simulink model "BMS_CurrentLimitsCalc_COM_Harness_MIL"  (R2022b)
settings: configuration reference "BMS_Sw_CodeGenConfig" (kept outside this file)
model workspace: external: MAT-File H:\0\New MAAM\10 - MBD\Battary Management System\SWE.3 CDD\DataTypes\Data_Script.mat (data not in the file)
undefined symbols (not defined in the file): BATT, Schedule
settings Model: DataDictionary=BMS_Arch_DD.sldd  Creator=MAAM  LastModifiedBy=MAAM
settings ConfigSetRef: SourceName=BMS_Sw_CodeGenConfig

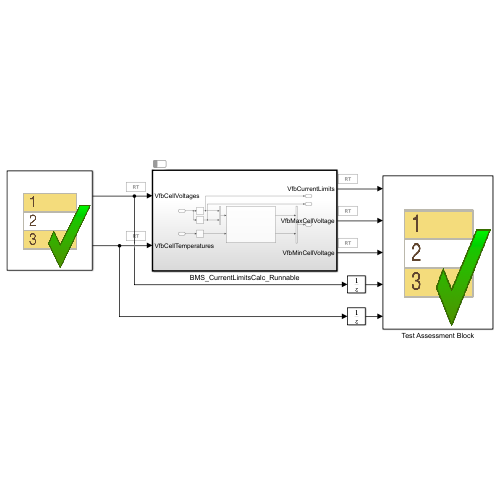
[thumbnail: Simulink's stored preview of the top-level diagram]
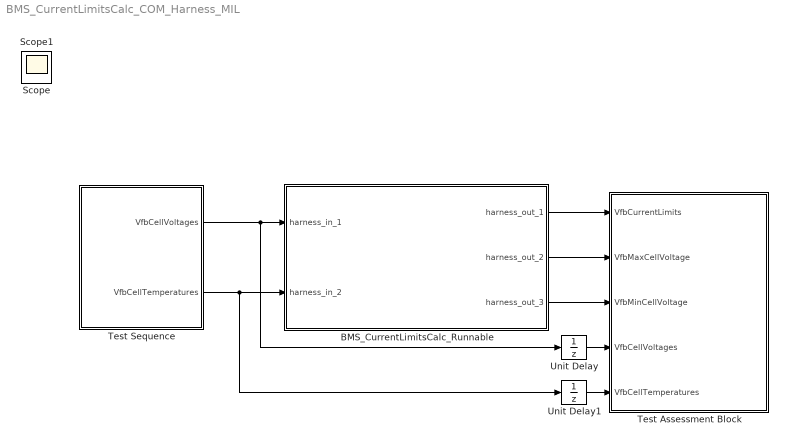
== system BMS_CurrentLimitsCalc_COM_Harness_MIL ==
  BMS_CurrentLimitsCalc_Runnable : Subsystem  Tag=__SL_testing_harness_stub_  Priority=0
  Test Assessment Block : Test Sequence  Tag=__SLT_ASMT__  TreatAsAtomicUnit=on  SystemSampleTime=Schedule.BMS_CurrentLimitsCalc_Task
  Test Sequence : Test Sequence  TreatAsAtomicUnit=on
  Unit Delay : UnitDelay  SampleTime=-1  HasFrameUpgradeWarning=on
  Unit Delay1 : UnitDelay  SampleTime=-1  HasFrameUpgradeWarning=on
  Scope : Scope
  Scope1 : Scope
  wires:
  Test Sequence/1(VfbCellVoltages) -> BMS_CurrentLimitsCalc_Runnable/1(harness_in_1), Unit Delay/1
  Test Sequence/2(VfbCellTemperatures) -> BMS_CurrentLimitsCalc_Runnable/2(harness_in_2), Unit Delay1/1
  BMS_CurrentLimitsCalc_Runnable/1(harness_out_1) -> Test Assessment Block/1(VfbCurrentLimits)
  BMS_CurrentLimitsCalc_Runnable/2(harness_out_2) -> Test Assessment Block/2(VfbMaxCellVoltage)
  BMS_CurrentLimitsCalc_Runnable/3(harness_out_3) -> Test Assessment Block/3(VfbMinCellVoltage)
  Unit Delay/1 -> Test Assessment Block/4(VfbCellVoltages)
  Unit Delay1/1 -> Test Assessment Block/5(VfbCellTemperatures)

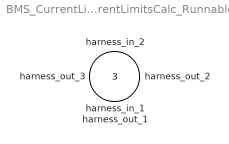
== system BMS_CurrentLimitsCalc_COM_Harness_MIL/BMS_CurrentLimitsCalc_Runnable ==
  harness_in_1 : Inport
  harness_in_2 : Inport  Port=2
  harness_out_1 : Outport
  harness_out_2 : Outport  Port=2
  harness_out_3 : Outport  Port=3

== stateflow chart BMS_CurrentLimitsCalc_COM_Harness_MIL/Test Assessment Block ==
  state Scenario_1
    state Run
      state Run_1
        verify(abs(VfbMaxCellVoltage - max(VfbCellVoltages)) <= tol);
        verify(abs(VfbMinCellVoltage  -  min(VfbCellVoltages)) <= tol);
        state Run_1_1
          if  (VfbMaxCellVoltage <= VMAXD) && (VfbMinCellVoltage >= VMIN) && (min(VfbCellTemperatures) <= TMIN)
          verify((VfbCurrentLimits(1) >= (-1.03 * ImaxDchrg)) && (VfbCurrentLimits(1) <= 0));
          end
          if  (VfbMaxCellVoltage <= VMAXC) && (VfbMinCellVoltage >= VMIN) && (min(VfbCellTemperatures) <= TMIN)
          verify((VfbCurrentLimits(2) <= ImaxChrg ) && (VfbCurrentLimits(2) >= 0));
          end
        (default) -> Run_1_1
      state Run_2
      (default) -> (junction 199)
      Run -> (junction 199)
      (junction 199) -> (junction 200) [order 1] : [t > 0
          | ]
      (junction 200) -> Run_1 [order 1] : [~in(Scenario_1.Run.Run_1)]
      (junction 200) -> (junction 203) [order 2]
      (junction 215) -> (junction 216)
      (junction 216) -> Run_2 [order 1] : [~in(Scenario_1.Run.Run_2)]
      (junction 216) -> (junction 219) [order 2]
      (junction 199) -> (junction 215) [order 2]
    (default) -> Run
  (default) -> Scenario_1 : {assert(Active_Scenario_Index == 1,'The value of Scenario Parameter ''Active_Scenario_Index'' is not valid. Use the index of the scenario to specify it.')}
  data: VfbCurrentLimits input single size=[2]; VfbMaxCellVoltage input single size=[1]; VfbMinCellVoltage input single size=[1]; VfbCellVoltages input single size=[BATT.Package.Ns_Module, BATT.Package.NumModules]; VfbCellTemperatures input single size=[BATT.Package.Ns_Module, BATT.Package.NumModules]; tol constant single =0.01; ImaxDchrg constant single size=1 =BATT.Current.Dchrg; ImaxChrg constant single size=1 =BATT.Current.Chrg; VMAXD constant single size=1 =BATT.Voltage.Full_Dchrg; VMIN parameter single size=1 =BATT.Voltage.Cut_off; TMIN constant single size=1 =max(BATT.Temperature.T_LUT); VMAXC parameter single size=1 =BATT.Voltage.Max_Chrg; Active_Scenario_Index parameter =1

== stateflow chart BMS_CurrentLimitsCalc_COM_Harness_MIL/Test Sequence ==
  settings: updateMethod=DISCRETE  sampleTime=0.1
  state StaticBoundary
    state S1
      Vs = ones(Ns, Num, 'single');
      Ts  = ones(Ns, Num, 'single');
      VfbCellVoltages = Vs * Vmin;
      VfbCellTemperatures = Ts * Tmin;
    state S2
      VfbCellVoltages = Vs * Vmax;
      VfbCellTemperatures = Ts * Tmin;
    state S3
      VfbCellVoltages = Vs * Vmin;
      VfbCellTemperatures = Ts * Tmax;
    state S4
      VfbCellVoltages = Vs * Vmax;
      VfbCellTemperatures = Ts * Tmax;
    state end
      coder.extrinsic('set_param');
      set_param(bdroot, 'SimulationCommand', 'stop');
    (default) -> StaticBoundary.S1
    StaticBoundary.S1 -> StaticBoundary.S2 : [
        | after(1, sec)
        | ]
    StaticBoundary.S2 -> StaticBoundary.S3 : [
        | after(1, sec)
        | ]
    StaticBoundary.S3 -> StaticBoundary.S4 : [
        | after(1, sec)
        | ]
    StaticBoundary.S4 -> StaticBoundary.end : [
        | after(1+1, sec)
        | ]
  state RandamTests
    state S1
      Vs = rand(Ns, Num, 'single');
      Ts  = rand(Ns, Num, 'single');
      VfbCellVoltages = Vs * Vmax;
      VfbCellTemperatures = (Ts * (Tmax - Tmin)) + Tmin;
    state S2
      Vs = rand(Ns, Num, 'single');
      Ts  = rand(Ns, Num, 'single');
      VfbCellVoltages = Vs * Vmax;
      VfbCellTemperatures = (Ts * (Tmax - Tmin)) + Tmin;
    state S3
      Vs = rand(Ns, Num, 'single');
      Ts  = rand(Ns, Num, 'single');
      VfbCellVoltages = Vs * Vmax;
      VfbCellTemperatures = (Ts * (Tmax - Tmin)) + Tmin;
    state S4
      Vs = rand(Ns, Num, 'single');
      Ts  = rand(Ns, Num, 'single');
      VfbCellVoltages = Vs * Vmax;
      VfbCellTemperatures = (Ts * (Tmax - Tmin)) + Tmin;
    state end
      coder.extrinsic('set_param');
      set_param(bdroot, 'SimulationCommand', 'stop');
    (default) -> RandamTests.S1
    RandamTests.S1 -> RandamTests.S2 : [
        | after(1, sec)
        | ]
    RandamTests.S2 -> RandamTests.S3 : [
        | after(1, sec)
        | ]
    RandamTests.S3 -> RandamTests.S4 : [
        | after(1, sec)
        | ]
    RandamTests.S4 -> RandamTests.end : [
        | after(1+1, sec)
        | ]
  state RampTests
    state Run
      Vs = ones(Ns, Num, 'single');
      Ts  = ones(Ns, Num, 'single');
      i = 1;
    state S1
      VfbCellVoltages = Vs * Vmin + (Vmax - Vmin) * ramp(et/5);
      VfbCellTemperatures = Ts * T_step(i);
      i = i + 1;
    state S2
    state S3
    state end
      coder.extrinsic('set_param');
      set_param(bdroot, 'SimulationCommand', 'stop');
    (default) -> Run
    Run -> RampTests.S1
    RampTests.S1 -> RampTests.S2
    RampTests.S2 -> RampTests.S1 [order 2] : [
        | after(5, sec)
        | ]
    RampTests.S2 -> RampTests.S3 [order 1] : [
        | i == length(T_step)
        | ]
    RampTests.S3 -> RampTests.end : [
        | after(5, sec)
        | ]
  (default) -> StaticBoundary [order 1] : [Active_Scenario_Index == 1]
  (default) -> RandamTests [order 2] : [Active_Scenario_Index == 2]
  (default) -> RampTests [order 3] : {assert(Active_Scenario_Index == 3,'The value of Scenario Parameter ''Active_Scenario_Index'' is not valid. Use the index of the scenario to specify it.')}
  data: VfbCellVoltages output single size=[BATT.Package.Ns_Module, BATT.Package.NumModules]; VfbCellTemperatures output single size=[BATT.Package.Ns_Module, BATT.Package.NumModules]; Active_Scenario_Index parameter =3; Vs local single size=[BATT.Package.Ns_Module, BATT.Package.NumModules]; Ts local single size=[BATT.Package.Ns_Module, BATT.Package.NumModules]; Ns constant single size=1 =BATT.Package.Ns_Module; Num constant single size=1 =BATT.Package.NumModules; Vmin constant single size=1 =VfbCellVoltages.Min; Vmax constant single size=1 =VfbCellVoltages.Max; Tmin constant single size=1 =VfbCellTemperatures.Min; Tmax constant single size=1 =VfbCellTemperatures.Max; T_step constant single size=size(BATT.Temperature.T_LUT) =BATT.Temperature.T_LUT; i local
